simulink model "ESTnew"  (R2025a)
settings: Solver=FixedStepAuto  StartTime=0.0  StopTime=stopt  FixedStep=deltat  MaxStep=0.05  RelTol=1e-3
InitFcn:
  | clear all;
  | close all;
  | clc;
  | 
  | % add the data and script directories
  | addpath('data','scripts');
  | 
  | % load the constants (units)
  | constants;
  | 
  | % load the simulation parameters
  | preprocessing;
StopFcn:
  | postprocessing;
values from neighbouring files (symbols this model uses):
  bStorage = 1e-6/unit("s")    [preprocessing.m]
  EStorageInitial = 2.0*unit("kWh")    [preprocessing.m]
  EStorageMax = 10.*unit("kWh")    [preprocessing.m]
  EStorageMin = 0.0*unit("kWh")    [preprocessing.m]
undefined symbols (not defined in the file or in its folder): etaTransformer, Length, LengthTwo, Rprime, V
settings Model: Creator=joche  LastModifiedBy=20244496
settings DataIOCC: SaveFormat=Array  SaveOutput=off  ReturnWorkspaceOutputs=off
settings OptimizationCC: ReuseModelBlockBuffer=off
settings ModelReferenceCC: EnableRefExpFcnMdlSchedulingChecks=on
settings RTWCC: GPUComputeCapability=3.5

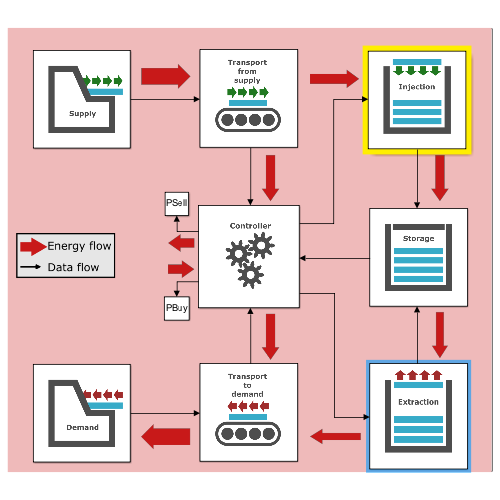
[thumbnail: Simulink's stored preview of the top-level diagram]
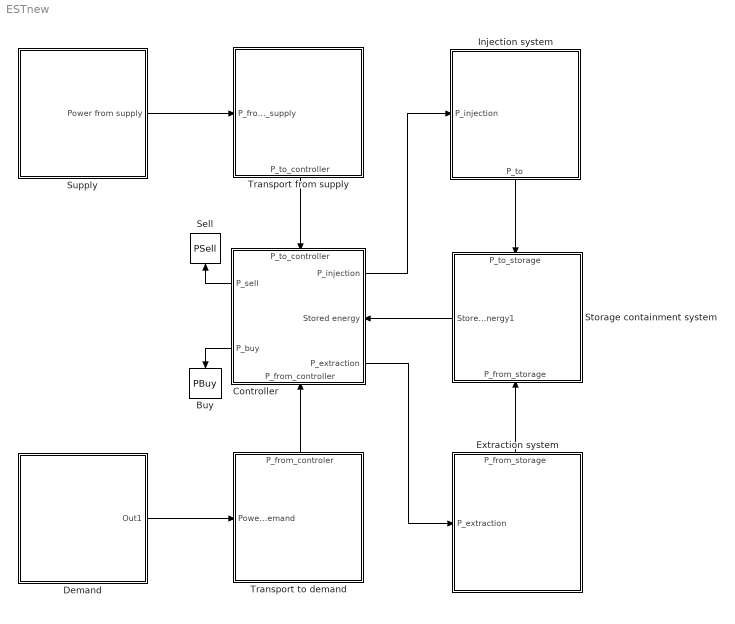
== system ESTnew ==
  Buy : ToWorkspace  VariableName=PBuy  SampleTime=-1
  Controller : Subsystem
      settings: PortSchema="{\"entries\":[{\"content\":{\"sides\":[{\"content\":{\"connectorIds\":[\"Out3\",\"Out4\"]},\"type\":\"ConnectorPlacement.EquallySpacedRectSide\",\"uuid\":\"4daf33ce-c96a-4783-b5c4-228eed953e01\"},{\"content\":{\"connectorIds\":[\"Out1\",\"In3\",\"Out2\"],\"side\":\"RIGHT\"},\"type\":\"ConnectorPlacement.EquallySpacedRectSide\",\"uuid\":\"e9942e50-8467-4af8-b79b-80636cbc76e5\"},{\"content\":{\"connectorIds\":[\"In1\"],\"side\":\"TOP\"},\"type\":\"ConnectorPlacement.EquallySpacedRectSide\",\"uuid\":\"f315e931-d69b-4751-b712-f89c6c81baeb\"},{\"content\":{\"connectorIds\":[\"In2\"],\"side\":\"BOTTOM\"},\"type\":\"ConnectorPlacement.EquallySpacedRectSide\",\"uuid\":\"44715ee6-5cd5-4669-bcb9-5ed7c869bdb3\"}]},\"type\":\"ConnectorPlacement.EquallySpacedConnector\",\"uuid\":\"fff48899-944b-4064-b7d7-ecc12144fb48\"}],\"packageUris\":[\"http://schema.mathworks.com/mf0/Connector/R2020b\"],\"version\":\"1.0\"}"
      mask Display: image('$imagefile'); % Use "Edit Image" on toolstrip to change.
  Demand : Subsystem
      mask Display: image('$imagefile'); % Use "Edit Image" on toolstrip to change.
  Extraction system : Subsystem
      settings: PortSchema="{\"entries\":[{\"content\":{\"sides\":[{\"content\":{},\"type\":\"ConnectorPlacement.EquallySpacedRectSide\",\"uuid\":\"05c5933d-55fc-4e06-853f-fc26d42905f9\"},{\"content\":{\"connectorIds\":[\"In1\"],\"side\":\"RIGHT\"},\"type\":\"ConnectorPlacement.EquallySpacedRectSide\",\"uuid\":\"327426c5-31d5-498b-a2bd-83e49353408c\"},{\"content\":{\"side\":\"TOP\"},\"type\":\"ConnectorPlacement.EquallySpacedRectSide\",\"uuid\":\"55306cf3-a3de-4385-a5ae-b8600ecdd5a2\"},{\"content\":{\"connectorIds\":[\"Out1\"],\"side\":\"BOTTOM\"},\"type\":\"ConnectorPlacement.EquallySpacedRectSide\",\"uuid\":\"08fcc9c3-40d3-4ac6-b914-dfeef6039ffb\"}]},\"type\":\"ConnectorPlacement.EquallySpacedConnector\",\"uuid\":\"cb35d5ba-e8c6-462c-b7b2-fe8356d4b0a1\"}],\"packageUris\":[\"http://schema.mathworks.com/mf0/Connector/R2020b\"],\"version\":\"1.0\"}"
      mask Display: image('$imagefile'); % Use "Edit Image" on toolstrip to change.
  Injection system : Subsystem
      settings: PortSchema="{\"entries\":[{\"content\":{\"sides\":[{\"content\":{\"connectorIds\":[]},\"type\":\"ConnectorPlacement.EquallySpacedRectSide\",\"uuid\":\"05c5933d-55fc-4e06-853f-fc26d42905f9\"},{\"content\":{\"connectorIds\":[\"In1\"],\"side\":\"RIGHT\"},\"type\":\"ConnectorPlacement.EquallySpacedRectSide\",\"uuid\":\"327426c5-31d5-498b-a2bd-83e49353408c\"},{\"content\":{\"connectorIds\":[\"Out1\"],\"side\":\"TOP\"},\"type\":\"ConnectorPlacement.EquallySpacedRectSide\",\"uuid\":\"55306cf3-a3de-4385-a5ae-b8600ecdd5a2\"},{\"content\":{\"connectorIds\":[],\"side\":\"BOTTOM\"},\"type\":\"ConnectorPlacement.EquallySpacedRectSide\",\"uuid\":\"08fcc9c3-40d3-4ac6-b914-dfeef6039ffb\"}]},\"type\":\"ConnectorPlacement.EquallySpacedConnector\",\"uuid\":\"cb35d5ba-e8c6-462c-b7b2-fe8356d4b0a1\"}],\"packageUris\":[\"http://schema.mathworks.com/mf0/Connector/R2020b\"],\"version\":\"1.0\"}"
      mask Display: image('$imagefile'); % Use "Edit Image" on toolstrip to change.
  Sell : ToWorkspace  VariableName=PSell  SampleTime=-1
  Storage containment system : Subsystem
      settings: PortSchema="{\"entries\":[{\"content\":{\"sides\":[{\"content\":{\"connectorIds\":[\"Out1\"]},\"type\":\"ConnectorPlacement.EquallySpacedRectSide\",\"uuid\":\"0ba48424-33b9-4934-970f-64fe5d8b070e\"},{\"content\":{\"connectorIds\":[],\"side\":\"RIGHT\"},\"type\":\"ConnectorPlacement.EquallySpacedRectSide\",\"uuid\":\"9cde340f-8f39-4499-9a12-5e1623737660\"},{\"content\":{\"connectorIds\":[\"In1\"],\"side\":\"TOP\"},\"type\":\"ConnectorPlacement.EquallySpacedRectSide\",\"uuid\":\"2af8db04-7fd0-4902-8637-8dc00edb4598\"},{\"content\":{\"connectorIds\":[\"In2\"],\"side\":\"BOTTOM\"},\"type\":\"ConnectorPlacement.EquallySpacedRectSide\",\"uuid\":\"e21ea806-d777-41a3-a53f-556fae66854b\"}]},\"type\":\"ConnectorPlacement.EquallySpacedConnector\",\"uuid\":\"4e2ddb36-4db3-4ab4-858b-ebb8ccefeb1f\"}],\"packageUris\":[\"http://schema.mathworks.com/mf0/Connector/R2020b\"],\"version\":\"1.0\"}"
      mask Display: image('$imagefile'); % Use "Edit Image" on toolstrip to change.
  Supply : Subsystem
      mask Display: image('$imagefile'); % Use "Edit Image" on toolstrip to change.
  Transport from supply : Subsystem
      settings: PortSchema="{\"entries\":[{\"content\":{\"sides\":[{\"content\":{\"connectorIds\":[\"In1\"]},\"type\":\"ConnectorPlacement.EquallySpacedRectSide\",\"uuid\":\"31329006-3d36-4d93-9c44-7503a515d397\"},{\"content\":{\"connectorIds\":[],\"side\":\"RIGHT\"},\"type\":\"ConnectorPlacement.EquallySpacedRectSide\",\"uuid\":\"aba139c7-f9b6-4881-a56b-a4cbbedacd88\"},{\"content\":{\"connectorIds\":[],\"side\":\"TOP\"},\"type\":\"ConnectorPlacement.EquallySpacedRectSide\",\"uuid\":\"e683eb73-7a35-4160-9c39-da83856a6278\"},{\"content\":{\"connectorIds\":[\"Out1\"],\"side\":\"BOTTOM\"},\"type\":\"ConnectorPlacement.EquallySpacedRectSide\",\"uuid\":\"1170dd18-447c-437f-9043-6812c2877331\"}]},\"type\":\"ConnectorPlacement.EquallySpacedConnector\",\"uuid\":\"804af608-1d70-444f-af69-e05f19bf98f3\"}],\"packageUris\":[\"http://schema.mathworks.com/mf0/Connector/R2020b\"],\"version\":\"1.0\"}"
      mask Display: image('$imagefile'); % Use "Edit Image" on toolstrip to change.
  Transport to demand : Subsystem
      settings: PortSchema="{\"entries\":[{\"content\":{\"sides\":[{\"content\":{\"connectorIds\":[\"In1\"]},\"type\":\"ConnectorPlacement.EquallySpacedRectSide\",\"uuid\":\"31329006-3d36-4d93-9c44-7503a515d397\"},{\"content\":{\"connectorIds\":[],\"side\":\"RIGHT\"},\"type\":\"ConnectorPlacement.EquallySpacedRectSide\",\"uuid\":\"aba139c7-f9b6-4881-a56b-a4cbbedacd88\"},{\"content\":{\"connectorIds\":[\"Out1\"],\"side\":\"TOP\"},\"type\":\"ConnectorPlacement.EquallySpacedRectSide\",\"uuid\":\"e683eb73-7a35-4160-9c39-da83856a6278\"},{\"content\":{\"connectorIds\":[],\"side\":\"BOTTOM\"},\"type\":\"ConnectorPlacement.EquallySpacedRectSide\",\"uuid\":\"c378138f-7233-4483-870c-40a69b3495ee\"}]},\"type\":\"ConnectorPlacement.EquallySpacedConnector\",\"uuid\":\"804af608-1d70-444f-af69-e05f19bf98f3\"}],\"packageUris\":[\"http://schema.mathworks.com/mf0/Connector/R2020b\"],\"version\":\"1.0\"}"
      mask Display: image('$imagefile'); % Use "Edit Image" on toolstrip to change.
  wires:
  Supply/1(Power from supply) -> Transport from supply/1(P_from_supply)
  Transport from supply/1(P_to_controller) -> Controller/1(P_to_controller)
  Transport to demand/1(P_from_controler) -> Controller/2(P_from_controller)
  Demand/1(Out1) -> Transport to demand/1(Power to demand)
  Controller/3(P_sell) -> Sell/1
  Controller/2(P_extraction) -> Extraction system/1(P_extraction)
  Injection system/1(P_to) -> Storage containment system/1(P_to_storage)
  Extraction system/1(P_from_storage) -> Storage containment system/2(P_from_storage)
  Storage containment system/1(Stored energy1) -> Controller/3(Stored energy)
  Controller/1(P_injection) -> Injection system/1(P_injection)
  Controller/4(P_buy) -> Buy/1

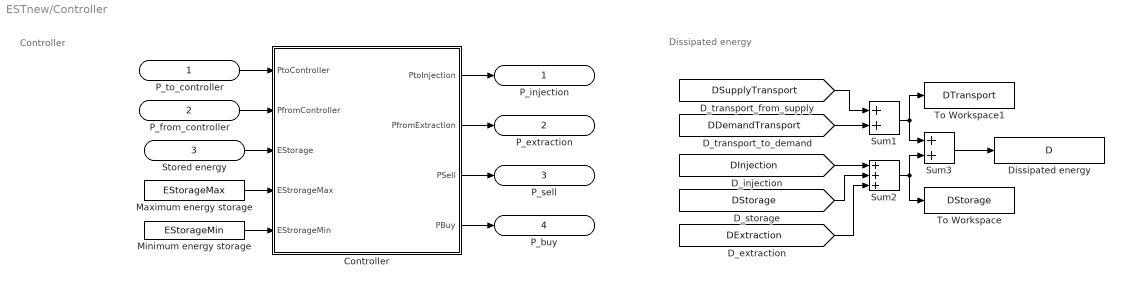
== system ESTnew/Controller ==
  note: Dissipated energy
  note: Controller
  P_to_controller : Inport
  P_from_controller : Inport  Port=2
  Stored energy : Inport  Port=3
  Controller : MATLAB Function  TreatAsAtomicUnit=on
  Dissipated energy : ToWorkspace  VariableName=D  SampleTime=-1
  Maximum energy storage : Constant  Value=EStorageMax
  Minimum energy storage : Constant  Value=EStorageMin
  Sum1 : Sum
  Sum2 : Sum  Inputs=+++
  Sum3 : Sum
  To Workspace : ToWorkspace  VariableName=DStorage  SampleTime=-1
  To Workspace1 : ToWorkspace  VariableName=DTransport  SampleTime=-1
  P_injection : Outport
  P_extraction : Outport  Port=2
  P_sell : Outport  Port=3
  P_buy : Outport  Port=4
  wires:
  P_from_controller/1 -> Controller/2(PfromController)
  Controller/2(PfromExtraction) -> P_extraction/1
  Controller/3(PSell) -> P_sell/1
  Controller/4(PBuy) -> P_buy/1
  Minimum energy storage/1 -> Controller/5(EStrorageMin)
  Maximum energy storage/1 -> Controller/4(EStrorageMax)
  P_to_controller/1 -> Controller/1(PtoController)
  Controller/1(PtoInjection) -> P_injection/1
  Stored energy/1 -> Controller/3(EStorage)
  [DDemandTransport] -> Sum1/2
  [DSupplyTransport] -> Sum1/1
  [DInjection] -> Sum2/1
  [DStorage] -> Sum2/2
  [DExtraction] -> Sum2/3
  Sum2/1 -> To Workspace/1, Sum3/2
  Sum1/1 -> To Workspace1/1, Sum3/1
  Sum3/1 -> Dissipated energy/1

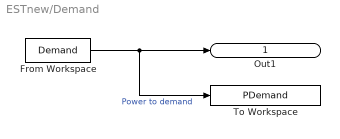
== system ESTnew/Demand ==
  From Workspace : FromWorkspace  VariableName=Demand  OutputAfterFinalValue=Setting to zero
  To Workspace : ToWorkspace  VariableName=PDemand  SampleTime=-1
  Out1 : Outport
  wires:
  From Workspace/1 -> To Workspace/1, Out1/1  "Power to demand"

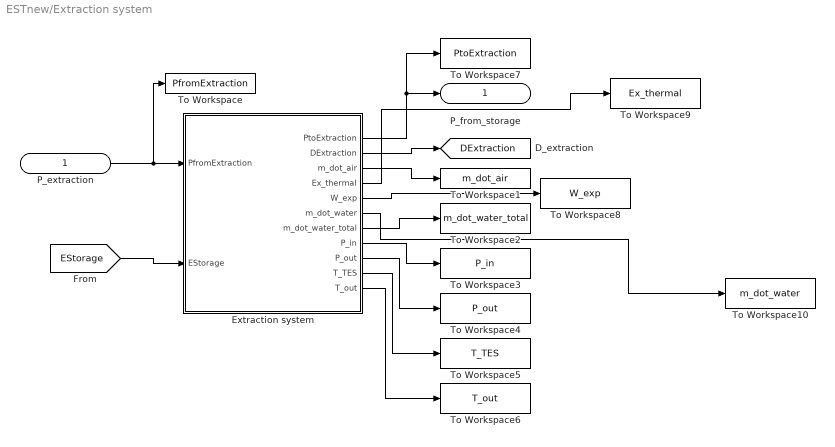
== system ESTnew/Extraction system ==
  P_extraction : Inport
  Extraction system : MATLAB Function  TreatAsAtomicUnit=on
  To Workspace : ToWorkspace  VariableName=PfromExtraction  SampleTime=-1
  To Workspace1 : ToWorkspace  VariableName=m_dot_air  SampleTime=-1
  To Workspace10 : ToWorkspace  VariableName=m_dot_water  SaveFormat=Timeseries  SampleTime=-1
  To Workspace2 : ToWorkspace  VariableName=m_dot_water_total  SaveFormat=Timeseries  SampleTime=-1
  To Workspace3 : ToWorkspace  VariableName=P_in  SaveFormat=Timeseries  SampleTime=-1
  To Workspace4 : ToWorkspace  VariableName=P_out  SaveFormat=Timeseries  SampleTime=-1
  To Workspace5 : ToWorkspace  VariableName=T_TES  SaveFormat=Timeseries  SampleTime=-1
  To Workspace6 : ToWorkspace  VariableName=T_out  SaveFormat=Timeseries  SampleTime=-1
  To Workspace7 : ToWorkspace  VariableName=PtoExtraction  SaveFormat=Timeseries  SampleTime=-1
  To Workspace8 : ToWorkspace  VariableName=W_exp  SaveFormat=Timeseries  SampleTime=-1
  To Workspace9 : ToWorkspace  VariableName=Ex_thermal  SaveFormat=Timeseries  SampleTime=-1
  P_from_storage : Outport
  tag scope: DExtraction=global
  wires:
  P_extraction/1 -> To Workspace/1, Extraction system/1(PfromExtraction)
  Extraction system/1(PtoExtraction) -> To Workspace7/1, P_from_storage/1
  Extraction system/2(DExtraction) -> [DExtraction]
  [EStorage] -> Extraction system/2(EStorage)
  Extraction system/3(m_dot_air) -> To Workspace1/1
  Extraction system/7(m_dot_water_total) -> To Workspace2/1
  Extraction system/8(P_in) -> To Workspace3/1
  Extraction system/9(P_out) -> To Workspace4/1
  Extraction system/10(T_TES) -> To Workspace5/1
  Extraction system/11(T_out) -> To Workspace6/1
  Extraction system/5(W_exp) -> To Workspace8/1
  Extraction system/4(Ex_thermal) -> To Workspace9/1
  Extraction system/6(m_dot_water) -> To Workspace10/1

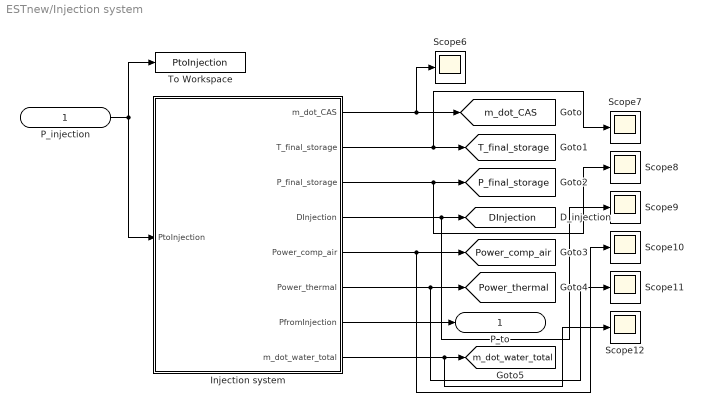
== system ESTnew/Injection system ==
  P_injection : Inport
  Injection system : MATLAB Function  TreatAsAtomicUnit=on
  Scope{6..12} (7 alike) : Scope
      Scope10 settings: ActiveDisplayYMinimum=-1  ActiveDisplayYMaximum=1  DataLoggingVariableName=ScopeData10
      Scope11 settings: ActiveDisplayYMinimum=-1  ActiveDisplayYMaximum=1  DataLoggingVariableName=ScopeData11
      Scope12 settings: ActiveDisplayYMinimum=-1  ActiveDisplayYMaximum=1  DataLoggingVariableName=ScopeData12
      Scope6 settings: ActiveDisplayYMinimum=-1  ActiveDisplayYMaximum=1  DataLoggingVariableName=ScopeData6
      Scope7 settings: ActiveDisplayYMinimum=-1  ActiveDisplayYMaximum=1  DataLoggingVariableName=ScopeData7
      Scope8 settings: ActiveDisplayYMinimum=-1  ActiveDisplayYMaximum=1  DataLoggingVariableName=ScopeData8
      Scope9 settings: ActiveDisplayYMinimum=-1  ActiveDisplayYMaximum=1  DataLoggingVariableName=ScopeData9
  To Workspace : ToWorkspace  VariableName=PtoInjection  SampleTime=-1
  P_to : Outport
  tag scope: DInjection=global, P_final_storage=global, Power_comp_air=global, Power_thermal=global, T_final_storage=global, m_dot_CAS=global, m_dot_water_total=global
  wires:
  P_injection/1 -> To Workspace/1, Injection system/1(PtoInjection)
  Injection system/7(PfromInjection) -> P_to/1
  Injection system/4(DInjection) -> Scope9/1, [DInjection]
  Injection system/1(m_dot_CAS) -> Scope6/1, [m_dot_CAS]
  Injection system/3(P_final_storage) -> Scope8/1, [P_final_storage]
  Injection system/2(T_final_storage) -> Scope7/1, [T_final_storage]
  Injection system/5(Power_comp_air) -> Scope10/1, [Power_comp_air]
  Injection system/6(Power_thermal) -> Scope11/1, [Power_thermal]
  Injection system/8(m_dot_water_total) -> Scope12/1, [m_dot_water_total]

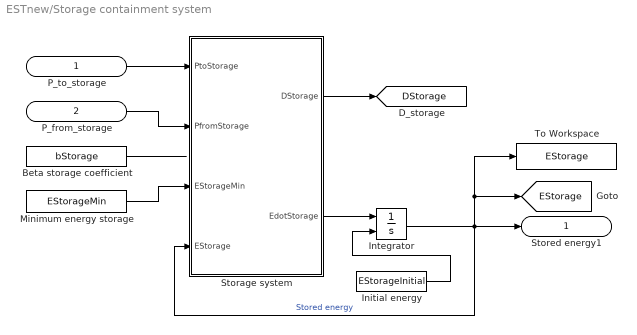
== system ESTnew/Storage containment system ==
  P_to_storage : Inport
  P_from_storage : Inport  Port=2
  Beta storage coefficient : Constant  Value=bStorage
  Initial energy : Constant  Value=EStorageInitial
  Integrator : Integrator  InitialConditionSource=external
  Minimum energy storage : Constant  Value=EStorageMin
  Storage system : MATLAB Function  TreatAsAtomicUnit=on
  To Workspace : ToWorkspace  VariableName=EStorage  SampleTime=-1
  Stored energy1 : Outport
  tag scope: DStorage=global, EStorage=global
  wires:
  P_from_storage/1 -> Storage system/2(PfromStorage)
  P_to_storage/1 -> Storage system/1(PtoStorage)
  Initial energy/1 -> Integrator/2
  Integrator/1 -> [EStorage], To Workspace/1, Storage system/4(EStorage), Stored energy1/1  "Stored energy"
  Storage system/1(DStorage) -> [DStorage]
  Beta storage coefficient/1 -> ?
  Storage system/2(EdotStorage) -> Integrator/1
  Minimum energy storage/1 -> Storage system/3(EStorageMin)

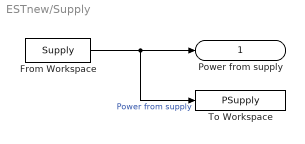
== system ESTnew/Supply ==
  From Workspace : FromWorkspace  VariableName=Supply  OutputAfterFinalValue=Setting to zero
  To Workspace : ToWorkspace  VariableName=PSupply  SampleTime=-1
  Power from supply : Outport
  wires:
  From Workspace/1 -> To Workspace/1, Power from supply/1  "Power from supply"

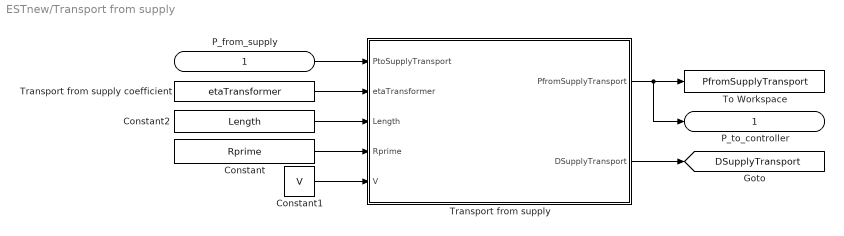
== system ESTnew/Transport from supply ==
  P_from_supply : Inport
  Constant : Constant  Value=Rprime
  Constant1 : Constant  Value=V
  Constant2 : Constant  Value=Length
  To Workspace : ToWorkspace  VariableName=PfromSupplyTransport  SampleTime=-1
  Transport from supply : MATLAB Function  TreatAsAtomicUnit=on
  Transport from supply coefficient : Constant  Value=etaTransformer
  P_to_controller : Outport
  tag scope: DSupplyTransport=global
  wires:
  Transport from supply coefficient/1 -> Transport from supply/2(etaTransformer)
  P_from_supply/1 -> Transport from supply/1(PtoSupplyTransport)
  Transport from supply/1(PfromSupplyTransport) -> P_to_controller/1, To Workspace/1
  Transport from supply/2(DSupplyTransport) -> [DSupplyTransport]
  Constant2/1 -> Transport from supply/3(Length)
  Constant/1 -> Transport from supply/4(Rprime)
  Constant1/1 -> Transport from supply/5(V)

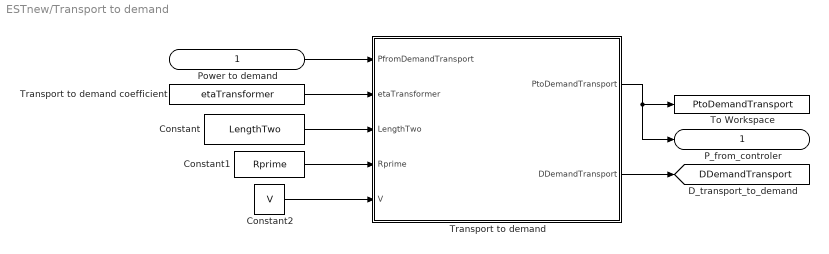
== system ESTnew/Transport to demand ==
  Power to demand : Inport
  Constant : Constant  Value=LengthTwo
  Constant1 : Constant  Value=Rprime
  Constant2 : Constant  Value=V
  To Workspace : ToWorkspace  VariableName=PtoDemandTransport  SampleTime=-1
  Transport to demand : MATLAB Function  TreatAsAtomicUnit=on
  Transport to demand coefficient : Constant  Value=etaTransformer
  P_from_controler : Outport
  tag scope: DDemandTransport=global
  wires:
  Transport to demand coefficient/1 -> Transport to demand/2(etaTransformer)
  Power to demand/1 -> Transport to demand/1(PfromDemandTransport)
  Transport to demand/1(PtoDemandTransport) -> P_from_controler/1, To Workspace/1
  Transport to demand/2(DDemandTransport) -> [DDemandTransport]
  Constant/1 -> Transport to demand/3(LengthTwo)
  Constant1/1 -> Transport to demand/4(Rprime)
  Constant2/1 -> Transport to demand/5(V)

== matlab function ESTnew/Transport to demand/Transport to demand ==
  data: PfromDemandTransport input; PtoDemandTransport output; etaTransformer input; DDemandTransport output; LengthTwo input; Rprime input; V input
function [PtoDemandTransport, DDemandTransport] = demandTransport(PfromDemandTransport, etaTransformer, LengthTwo, Rprime, V)
    PtoDemandTransport = (etaTransformer^2) * PfromDemandTransport - (etaTransformer^3) * LengthTwo * Rprime * (PfromDemandTransport/V)^2;
    DDemandTransport = PfromDemandTransport - PtoDemandTransport;  % Losses
end

== matlab function ESTnew/Injection system/Injection system ==
  data: m_dot_CAS output; T_final_storage output; P_final_storage output; DInjection output; Power_comp_air output; Power_thermal output; PtoInjection input; PfromInjection output; m_dot_water_total output
function [m_dot_CAS, T_final_storage, P_final_storage, DInjection, Power_comp_air, Power_thermal, PfromInjection, m_dot_water_total] = injection(PtoInjection)
%% ==== MULTI-STAGE COMPRESSION AND COOLING SYSTEM WITH LOOP =====
%% === Constants ===
   n = 1.4;                          % Adiabatic index for air
   eta_comp_motor = 0.9;            % Compressor motor efficiency
   eta_isentropic_comp = 0.9;       % Isentropic efficiency of compressor
   cp_air = 1005;                   % Specific heat capacity of air [J/kg.K]
   cp_water = 4180;                 % Specific heat capacity of water [J/kg.K]
   epsilon_HX = 0.7;                % Heat exchanger effectiveness
   R_air = 287;                     % Gas constant for air [J/kg.K]
   T_atm = 290;                     % Ambient temperature [K]
   P_atm = 1e5;                     % Atmospheric pressure [Pa]
   T_coolant_in = 333;             % Coolant inlet temperature [K]
   T_water_max = 453;              % Max water temperature for cooling [K]
   
%% === Stage pressures ===
   P_stage = [8e5, 20e5, 45e5];

%% === Initialize arrays ===
   T_in = zeros(1,4); T_out = zeros(1,3); T_HX = zeros(1,3);
   P_in = zeros(1,4); P_out = zeros(1,3); P_HX = zeros(1,3);
   specific_work = zeros(1,3); Power_thermal_i = zeros(1,3);
   m_dot_water = zeros(1,3);
   
   T_in(1) = T_atm;
   P_in(1) = P_atm;

%% === Loop over stages ===
   for i = 1:3
       % Isentropic temperature
       T_isentropic = T_in(i) * (P_stage(i) / P_in(i))^((n - 1) / n);
       
       % Compressor outlet temperature
       T_out(i) = T_in(i) + (T_isentropic - T_in(i)) / eta_isentropic_comp;
       
       % After heat exchanger temperature
       T_HX(i) = T_out(i) - epsilon_HX * (T_out(i) - T_coolant_in);
       
       % After heat exchanger pressure
       P_out(i) = P_stage(i);
       P_HX(i) = P_out(i) * (T_HX(i) / T_out(i));
       
       % Specific work
       specific_work(i) = cp_air * (T_out(i) - T_in(i));
       
       % Exergy loss (thermal power removed)
       Ex_thermal = cp_air * ((T_out(i) - T_atm) - T_atm * log(T_out(i)/T_atm)) ...
                  - cp_air * ((T_HX(i) - T_atm) - T_atm * log(T_HX(i)/T_atm));
       Power_thermal_i(i) = Ex_thermal; % Still in W, converted later
       
       % Prepare next stage input
       T_in(i+1) = T_HX(i);
       P_in(i+1) = P_HX(i);
   end

%% === Total Power and Mass Flow ===
   total_specific_work = sum(specific_work);
   m_dot_CAS = (PtoInjection * 1000 * eta_comp_motor) / total_specific_work;
   T_final_storage = T_HX(end);
   P_final_storage = P_HX(end);

   % Power required for compressing air (in kW)
   Power_comp_air = m_dot_CAS * (cp_air * (T_final_storage - T_atm) ...
       - T_atm * (cp_air * log(T_final_storage / T_atm) - R_air * log(P_final_storage / P_atm))) / 1000;

   % Total thermal exergy loss (in kW)
   Power_thermal_i = m_dot_CAS * Power_thermal_i / 1000; 
   Power_thermal = sum(Power_thermal_i);

   % Power accounting
   PfromInjection = Power_comp_air + Power_thermal;
   DInjection = PtoInjection - PfromInjection;

%% === Cooling water flow rates ===
   for i = 1:3
       m_dot_water(i) = (Power_thermal_i(i) * 1000) / (cp_water * (T_water_max - T_coolant_in));
   end
   m_dot_water_total = sum(m_dot_water);
end

== matlab function ESTnew/Transport from supply/Transport from supply ==
  data: PtoSupplyTransport input; PfromSupplyTransport output; etaTransformer input; DSupplyTransport output; Length input; Rprime input; V input
function [PfromSupplyTransport, DSupplyTransport] = supplyTransport(PtoSupplyTransport, etaTransformer, Length, Rprime, V)
    % Modelling for the power lines and transformers
    L = Length;
    PfromSupplyTransport = (etaTransformer^2)*PtoSupplyTransport - (etaTransformer^3)*L*Rprime*(PtoSupplyTransport/V)^2;
    DSupplyTransport = PtoSupplyTransport - PfromSupplyTransport;
end

== matlab function ESTnew/Controller/Controller ==
  data: PtoInjection output; PfromExtraction output; PSell output; PBuy output; PtoController input; PfromController input; EStorage input; EStrorageMax input; EStrorageMin input
function [PtoInjection, PfromExtraction, PSell, PBuy] = controller(PtoController, PfromController, EStorage, EStrorageMax, EStrorageMin)
    
    %% Power surplus or deficit

    deltaP = PtoController - PfromController;

    % Power surplus
    if deltaP >= 0

        %% Storage injection

        % Storage system is not full
        if EStorage < EStrorageMax 

            PtoInjection = deltaP;

        % Storage system is full
        else
            PtoInjection = 0;
        end

        %% Storage extraction

        PfromExtraction = 0;

        %% Load-balancing
        PSell   = deltaP - PtoInjection;
        PBuy    = 0;

    % Power deficit
    else

        %% Storage injection

        PtoInjection = 0;

        %% Storage extraction

        % Storage system is not empty
        if EStorage > EStrorageMin

            PfromExtraction = -deltaP;

        % Storage system is empty
        else
            PfromExtraction = 0;
        end

        %% Load-balancing

        PSell = 0;
        PBuy  = -deltaP - PfromExtraction;
    end

== matlab function ESTnew/Extraction system/Extraction system ==
  data: PfromExtraction input; PtoExtraction output; DExtraction output; EStorage input; m_dot_air output; Ex_thermal output; W_exp output; m_dot_water output; m_dot_water_total output; P_in output; P_out output; T_TES output; T_out output
function [PtoExtraction, DExtraction, m_dot_air,Ex_thermal, W_exp,  m_dot_water,m_dot_water_total, P_in, P_out, T_TES, T_out] = extraction(PfromExtraction, EStorage)
    %% MULTISTAGE AIR EXPANSION SYSTEM - STANDALONE TEST SCRIPT
    % Simulates a 3-stage air expansion system with inter-stage reheating.
    % Calculates: 
    % - Mechanical work extracted from each stage
    % - Thermal exergy drawn from TES
    % - Cooling water requirements for reheating
    % - Overall power delivered to the building
    % - Pressure & temperature evolution across stages

    %% ===================== PHYSICAL CONSTANTS =====================
    cp_air = 1005;      % [J/kg·K] Specific heat capacity of air
    cp_water = 4180;    % [J/kg·K] Specific heat of water
    eta_turbine = 0.88; % [-] Isentropic efficiency of the air turbine
    n = 1.4;            % [-] Polytropic index for dry air
    T0 = 290;           % [K] Ambient/reference temperature (final desired output temp)

    %% ===================== SYSTEM INPUTS ==========================
    %%PfromExtraction = 7000;         % [kW] Power demand to be covered from storage
    %% E_CAS = 3.2e9;                  % [J] Available energy in Compressed Air Storage (CAS)

    % Reheat temperatures after each expansion stage from TES (or constant for now)
    T_TES = [550, 520, 510];        % [K]

    % Stage-wise pressure conditions
    P_in = [30e5, 25e5, 10e5];      % [Pa] Inlet pressures before each expansion stage
    P_out = [25e5, 10e5, 1e5];      % [Pa] Outlet pressures after each expansion stage

    %% ============== INITIALIZE OUTPUT VARIABLES ===================
    W_exp = zeros(1,3);         % [J/kg] Work recovered per stage
    Ex_thermal = zeros(1,3);    % [J/kg] Thermal exergy used for reheating
    T_out = zeros(1,3);         % [K] Outlet temperatures after expansion
    m_dot_water = zeros(1,3);   % [kg/s] Water flow rate per stage for reheating

    %% ============== PER-STAGE THERMODYNAMICS ======================
    for i = 1:3
        % Ideal isentropic outlet temperature
        T_isentropic = T_TES(i) * (P_out(i) / P_in(i)) ^ ((n - 1) / n);
    
        % Real outlet temperature with turbine inefficiency
        T_out(i) = T_TES(i) - (T_TES(i) - T_isentropic) * eta_turbine;

        % Specific work output per kg of air
        W_exp(i) = cp_air * (T_TES(i) - T_out(i));

        % Thermal exergy input from TES
        Ex_in = cp_air * (T_TES(i) - T0) - T0 * cp_air * log(T_TES(i) / T0);
        Ex_thermal(i) = Ex_in;

        % Required water mass flow for reheating at each stage
        deltaT = T_TES(i) - T0;
        m_dot_water(i) = (cp_air * deltaT) / (cp_water * deltaT);  % Simplifies to cp_air / cp_water
    end

    %% ============== SYSTEM-LEVEL CALCULATIONS =====================
    W_exp_total = sum(W_exp);              % [J/kg] Total work extractable per kg
    Ex_total_per_kg = sum(Ex_thermal);     % [J/kg] Total thermal exergy input per kg
    m_dot_water_total = sum(m_dot_water);  % [kg/s] Total water mass flow across all stages

    % Calculate maximum allowable air mass flow based on CAS energy
    max_m_dot_air = EStorage / Ex_total_per_kg;

    % Required air mass flow to meet building power demand
    required_m_dot_air = (PfromExtraction * 1000) / W_exp_total;

    % Compare required vs available air mass flow
    if required_m_dot_air <= max_m_dot_air
        % Sufficient CAS energy to fully meet demand
        m_dot_air = required_m_dot_air;
        PtoExtraction = PfromExtraction;
        DExtraction = 0;
    else
        % Insufficient CAS energy: partial supply, rest from grid
        m_dot_air = max_m_dot_air;
        PtoExtraction = m_dot_air * W_exp_total / 1000;  % Actual deliverable power [kW]
        DExtraction = PfromExtraction - PtoExtraction;   % Shortfall [kW]
    end

== matlab function ESTnew/Storage containment system/Storage system ==
  data: DStorage output; EdotStorage output; PtoStorage input; PfromStorage input; EStorageMin input; EStorage input
function [DStorage, EdotStorage]= Storage(PtoStorage, PfromStorage, EStorageMin, EStorage)
    %% === Constants ===
   r_tank = 1.43;    % Outer radius of tank for compressed air[m]
   L_tank = 6.50;    % Length of tank [m]
   r_TES = 3.00;     % Inner radius of thermal tank [m]
   H_TES = 8.24;     % Height of thermal tank [m]
   t_ins_CAES         = 0.10;    % CAES Insulation thickness [m]
   k_ins_CAES         = 0.002;   % CAES Insulation  thermal conductivity [W/(m*K)]
   t_ins_TES     = 0.10;    % TES Insulation thickness [m]
   k_ins_TES     = 0.07;    % TES Insulation thermal conductivity [W/(m*K)]
   m_air         = 1.48e3;  % Mass of compressed air in CAES tank[kg]
   c_air        = 1.005;   % Specific heat capacity of air [J/(kg*K)]
   m_salt        = 4.20e5;  % Mass of molten salt in TES tank[kg]
   c_salt       = 1500;    % Specific heat capacity of molten salt [J/(kg*K)]
%% === Dissipation coefficient calculation ===
   R_cond_CAES = log((r_tank + t_ins_CAES ) ./ r_tank) ...
                ./ (2 * pi * k_ins_CAES * L_tank);
   R_cond_TES = log((r_TES + t_ins_TES ) ./ r_TES) ...
                ./ (2 * pi * k_ins_TES * H_TES);
   R_tot = R_cond_CAES * R_cond_TES / (R_cond_TES + R_cond_CAES);
   Heat_capacity_CAES = m_air * c_air;
   Heat_capacity_TES = m_salt * c_salt;
   Heat_capacity_tot = Heat_capacity_CAES + Heat_capacity_TES;
   bStorage = 1 / (Heat_capacity_tot * R_tot);
%% === Dissipated power & Power in the storage ===
   DStorage = bStorage * (EStorage-EStorageMin);
   EdotStorage = PtoStorage - PfromStorage - DStorage;
